simulink library "mbd_s32k_examples"  (Simulink 9.0)
settings: Solver=FixedStepDiscrete  StartTime=0.0  StopTime=10.0  FixedStep=0.1  RelTol=1e-3  EnableMultiTasking=on
InitFcn:
  | mbd_s32k14_consistency_checks(bdroot(gcs));
(part 3 of 3)

== system mbd_s32k_examples/S32K11x MCU Simulink Models/Communications Modules/CAN/CAN_Loopback ==
  Gain : Gain  SaturateOnIntegerOverflow=on  OutDataTypeStr=Inherit: Same as input  ParamDataTypeStr=Inherit: Same as input

== system mbd_s32k_examples/S32K11x MCU Simulink Models/Communications Modules/CAN/CAN_Master_XFER ==
  Gain : Gain  SaturateOnIntegerOverflow=on  OutDataTypeStr=Inherit: Same as input  ParamDataTypeStr=Inherit: Same as input

== system mbd_s32k_examples/S32K11x MCU Simulink Models/Communications Modules/CAN/CAN_Traffic ==
  Gain : Gain  SaturateOnIntegerOverflow=on  OutDataTypeStr=Inherit: Same as input  ParamDataTypeStr=Inherit: Same as input

== system mbd_s32k_examples/S32K11x MCU Simulink Models/Communications Modules/FlexIO/FlexIO_I2C_Master_RX ==
  Gain : Gain  SaturateOnIntegerOverflow=on  OutDataTypeStr=Inherit: Same as input  ParamDataTypeStr=Inherit: Same as input

== system mbd_s32k_examples/S32K11x MCU Simulink Models/Communications Modules/FlexIO/FlexIO_I2C_Master_TX ==
  Gain : Gain  SaturateOnIntegerOverflow=on  OutDataTypeStr=Inherit: Same as input  ParamDataTypeStr=Inherit: Same as input

== system mbd_s32k_examples/S32K11x MCU Simulink Models/Communications Modules/FlexIO/FlexIO_I2C_Slave_RX ==
  Gain : Gain  SaturateOnIntegerOverflow=on  OutDataTypeStr=Inherit: Same as input  ParamDataTypeStr=Inherit: Same as input

== system mbd_s32k_examples/S32K11x MCU Simulink Models/Communications Modules/FlexIO/FlexIO_I2C_Slave_TX ==
  Gain : Gain  SaturateOnIntegerOverflow=on  OutDataTypeStr=Inherit: Same as input  ParamDataTypeStr=Inherit: Same as input

== system mbd_s32k_examples/S32K11x MCU Simulink Models/Communications Modules/FlexIO/FlexIO_SPI_Master_TX ==
  Gain : Gain  SaturateOnIntegerOverflow=on  OutDataTypeStr=Inherit: Same as input  ParamDataTypeStr=Inherit: Same as input

== system mbd_s32k_examples/S32K11x MCU Simulink Models/Communications Modules/FlexIO/FlexIO_SPI_Slave_TX ==
  Gain : Gain  SaturateOnIntegerOverflow=on  OutDataTypeStr=Inherit: Same as input  ParamDataTypeStr=Inherit: Same as input

== system mbd_s32k_examples/S32K11x MCU Simulink Models/Communications Modules/FlexIO/FlexIO_UART_RX ==
  Gain : Gain  SaturateOnIntegerOverflow=on  OutDataTypeStr=Inherit: Same as input  ParamDataTypeStr=Inherit: Same as input

== system mbd_s32k_examples/S32K11x MCU Simulink Models/Communications Modules/FlexIO/FlexIO_UART_TX ==
  Gain : Gain  SaturateOnIntegerOverflow=on  OutDataTypeStr=Inherit: Same as input  ParamDataTypeStr=Inherit: Same as input

== system mbd_s32k_examples/S32K11x MCU Simulink Models/Communications Modules/I2C/I2C_Master_Request ==
  Gain : Gain  SaturateOnIntegerOverflow=on  OutDataTypeStr=Inherit: Same as input  ParamDataTypeStr=Inherit: Same as input

== system mbd_s32k_examples/S32K11x MCU Simulink Models/Communications Modules/I2C/I2C_Master_Send ==
  Gain : Gain  SaturateOnIntegerOverflow=on  OutDataTypeStr=Inherit: Same as input  ParamDataTypeStr=Inherit: Same as input

== system mbd_s32k_examples/S32K11x MCU Simulink Models/Communications Modules/I2C/I2C_Slave_Receive ==
  Gain : Gain  SaturateOnIntegerOverflow=on  OutDataTypeStr=Inherit: Same as input  ParamDataTypeStr=Inherit: Same as input

== system mbd_s32k_examples/S32K11x MCU Simulink Models/Communications Modules/I2C/I2C_Slave_Send ==
  Gain : Gain  SaturateOnIntegerOverflow=on  OutDataTypeStr=Inherit: Same as input  ParamDataTypeStr=Inherit: Same as input

== system mbd_s32k_examples/S32K11x MCU Simulink Models/Communications Modules/SPI/SPI_Master_Slave_Communication ==
  Gain : Gain  SaturateOnIntegerOverflow=on  OutDataTypeStr=Inherit: Same as input  ParamDataTypeStr=Inherit: Same as input

== system mbd_s32k_examples/S32K11x MCU Simulink Models/Communications Modules/Serial/UART_Echo ==
  Gain : Gain  SaturateOnIntegerOverflow=on  OutDataTypeStr=Inherit: Same as input  ParamDataTypeStr=Inherit: Same as input

== system mbd_s32k_examples/S32K11x MCU Simulink Models/Communications Modules/Serial/UART_Hello_World ==
  Gain : Gain  SaturateOnIntegerOverflow=on  OutDataTypeStr=Inherit: Same as input  ParamDataTypeStr=Inherit: Same as input

== system mbd_s32k_examples/S32K14x MCU Simulink Models/AMMCLIB/AMCLIB/AMCLIB_BackEMF_OBSERVER_F16 ==
  Gain : Gain  SaturateOnIntegerOverflow=on  OutDataTypeStr=Inherit: Same as input  ParamDataTypeStr=Inherit: Same as input

== system mbd_s32k_examples/S32K14x MCU Simulink Models/AMMCLIB/AMCLIB/AMCLIB_BackEMF_OBSERVER_F32 ==
  Gain : Gain  SaturateOnIntegerOverflow=on  OutDataTypeStr=Inherit: Same as input  ParamDataTypeStr=Inherit: Same as input

== system mbd_s32k_examples/S32K14x MCU Simulink Models/AMMCLIB/AMCLIB/AMCLIB_BackEMF_OBSERVER_FLT ==
  Gain : Gain  SaturateOnIntegerOverflow=on  OutDataTypeStr=Inherit: Same as input  ParamDataTypeStr=Inherit: Same as input

== system mbd_s32k_examples/S32K14x MCU Simulink Models/AMMCLIB/AMCLIB/AMCLIB_CURRENT_LOOP ==
  Gain : Gain  SaturateOnIntegerOverflow=on  OutDataTypeStr=Inherit: Same as input  ParamDataTypeStr=Inherit: Same as input

== system mbd_s32k_examples/S32K14x MCU Simulink Models/AMMCLIB/AMCLIB/AMCLIB_FW ==
  Gain : Gain  SaturateOnIntegerOverflow=on  OutDataTypeStr=Inherit: Same as input  ParamDataTypeStr=Inherit: Same as input

== system mbd_s32k_examples/S32K14x MCU Simulink Models/AMMCLIB/AMCLIB/AMCLIB_SPEED_LOOP ==
  Gain : Gain  SaturateOnIntegerOverflow=on  OutDataTypeStr=Inherit: Same as input  ParamDataTypeStr=Inherit: Same as input

== system mbd_s32k_examples/S32K14x MCU Simulink Models/AMMCLIB/AMCLIB/AMCLIB_SPEED_LOOP_with_FW ==
  Gain : Gain  SaturateOnIntegerOverflow=on  OutDataTypeStr=Inherit: Same as input  ParamDataTypeStr=Inherit: Same as input

== system mbd_s32k_examples/S32K14x MCU Simulink Models/AMMCLIB/GDFLIB/GDFLIB_FIR ==
  Gain : Gain  SaturateOnIntegerOverflow=on  OutDataTypeStr=Inherit: Same as input  ParamDataTypeStr=Inherit: Same as input

== system mbd_s32k_examples/S32K14x MCU Simulink Models/AMMCLIB/GDFLIB/GDFLIB_IIR1 ==
  Gain : Gain  SaturateOnIntegerOverflow=on  OutDataTypeStr=Inherit: Same as input  ParamDataTypeStr=Inherit: Same as input

== system mbd_s32k_examples/S32K14x MCU Simulink Models/AMMCLIB/GDFLIB/GDFLIB_IIR2 ==
  Gain : Gain  SaturateOnIntegerOverflow=on  OutDataTypeStr=Inherit: Same as input  ParamDataTypeStr=Inherit: Same as input

== system mbd_s32k_examples/S32K14x MCU Simulink Models/AMMCLIB/GDFLIB/GDFLIB_MA ==
  Gain : Gain  SaturateOnIntegerOverflow=on  OutDataTypeStr=Inherit: Same as input  ParamDataTypeStr=Inherit: Same as input

== system mbd_s32k_examples/S32K14x MCU Simulink Models/AMMCLIB/GFLIB/GFLIB_LIMIT ==
  Gain : Gain  SaturateOnIntegerOverflow=on  OutDataTypeStr=Inherit: Same as input  ParamDataTypeStr=Inherit: Same as input

== system mbd_s32k_examples/S32K14x MCU Simulink Models/AMMCLIB/GFLIB/GFLIB_LOG ==
  Gain : Gain  SaturateOnIntegerOverflow=on  OutDataTypeStr=Inherit: Same as input  ParamDataTypeStr=Inherit: Same as input

== system mbd_s32k_examples/S32K14x MCU Simulink Models/AMMCLIB/GFLIB/GFLIB_LUT ==
  Gain : Gain  SaturateOnIntegerOverflow=on  OutDataTypeStr=Inherit: Same as input  ParamDataTypeStr=Inherit: Same as input

== system mbd_s32k_examples/S32K14x MCU Simulink Models/AMMCLIB/GFLIB/GFLIB_MISCELLANEOUS ==
  Gain : Gain  SaturateOnIntegerOverflow=on  OutDataTypeStr=Inherit: Same as input  ParamDataTypeStr=Inherit: Same as input

== system mbd_s32k_examples/S32K14x MCU Simulink Models/AMMCLIB/GFLIB/GFLIB_PIP ==
  Gain : Gain  SaturateOnIntegerOverflow=on  OutDataTypeStr=Inherit: Same as input  ParamDataTypeStr=Inherit: Same as input

== system mbd_s32k_examples/S32K14x MCU Simulink Models/AMMCLIB/GFLIB/GFLIB_PIR ==
  Gain : Gain  SaturateOnIntegerOverflow=on  OutDataTypeStr=Inherit: Same as input  ParamDataTypeStr=Inherit: Same as input

== system mbd_s32k_examples/S32K14x MCU Simulink Models/AMMCLIB/GFLIB/GFLIB_TRIGONOMETRIC ==
  Gain : Gain  SaturateOnIntegerOverflow=on  OutDataTypeStr=Inherit: Same as input  ParamDataTypeStr=Inherit: Same as input

== system mbd_s32k_examples/S32K14x MCU Simulink Models/AMMCLIB/GMCLIB/GMCLIB_FOC_F16 ==
  Gain : Gain  SaturateOnIntegerOverflow=on  OutDataTypeStr=Inherit: Same as input  ParamDataTypeStr=Inherit: Same as input

== system mbd_s32k_examples/S32K14x MCU Simulink Models/AMMCLIB/GMCLIB/GMCLIB_FOC_F32 ==
  Gain : Gain  SaturateOnIntegerOverflow=on  OutDataTypeStr=Inherit: Same as input  ParamDataTypeStr=Inherit: Same as input

== system mbd_s32k_examples/S32K14x MCU Simulink Models/AMMCLIB/GMCLIB/GMCLIB_FOC_FLT ==
  Gain : Gain  SaturateOnIntegerOverflow=on  OutDataTypeStr=Inherit: Same as input  ParamDataTypeStr=Inherit: Same as input

== system mbd_s32k_examples/S32K14x MCU Simulink Models/AMMCLIB/MLIB/MLIB_ABS ==
  Gain : Gain  SaturateOnIntegerOverflow=on  OutDataTypeStr=Inherit: Same as input  ParamDataTypeStr=Inherit: Same as input

== system mbd_s32k_examples/S32K14x MCU Simulink Models/AMMCLIB/MLIB/MLIB_ADD ==
  Gain : Gain  SaturateOnIntegerOverflow=on  OutDataTypeStr=Inherit: Same as input  ParamDataTypeStr=Inherit: Same as input

== system mbd_s32k_examples/S32K14x MCU Simulink Models/AMMCLIB/MLIB/MLIB_CONVERT ==
  Gain : Gain  SaturateOnIntegerOverflow=on  OutDataTypeStr=Inherit: Same as input  ParamDataTypeStr=Inherit: Same as input

== system mbd_s32k_examples/S32K14x MCU Simulink Models/AMMCLIB/MLIB/MLIB_DIV ==
  Gain : Gain  SaturateOnIntegerOverflow=on  OutDataTypeStr=Inherit: Same as input  ParamDataTypeStr=Inherit: Same as input

== system mbd_s32k_examples/S32K14x MCU Simulink Models/AMMCLIB/MLIB/MLIB_MAC ==
  Gain : Gain  SaturateOnIntegerOverflow=on  OutDataTypeStr=Inherit: Same as input  ParamDataTypeStr=Inherit: Same as input

== system mbd_s32k_examples/S32K14x MCU Simulink Models/AMMCLIB/MLIB/MLIB_MUL ==
  Gain : Gain  SaturateOnIntegerOverflow=on  OutDataTypeStr=Inherit: Same as input  ParamDataTypeStr=Inherit: Same as input

== system mbd_s32k_examples/S32K14x MCU Simulink Models/AMMCLIB/MLIB/MLIB_NEGATE ==
  Gain : Gain  SaturateOnIntegerOverflow=on  OutDataTypeStr=Inherit: Same as input  ParamDataTypeStr=Inherit: Same as input

== system mbd_s32k_examples/S32K14x MCU Simulink Models/AMMCLIB/MLIB/MLIB_NORM ==
  Gain : Gain  SaturateOnIntegerOverflow=on  OutDataTypeStr=Inherit: Same as input  ParamDataTypeStr=Inherit: Same as input

== system mbd_s32k_examples/S32K14x MCU Simulink Models/AMMCLIB/MLIB/MLIB_RND ==
  Gain : Gain  SaturateOnIntegerOverflow=on  OutDataTypeStr=Inherit: Same as input  ParamDataTypeStr=Inherit: Same as input

== system mbd_s32k_examples/S32K14x MCU Simulink Models/AMMCLIB/MLIB/MLIB_SHBI ==
  Gain : Gain  SaturateOnIntegerOverflow=on  OutDataTypeStr=Inherit: Same as input  ParamDataTypeStr=Inherit: Same as input

== system mbd_s32k_examples/S32K14x MCU Simulink Models/AMMCLIB/MLIB/MLIB_SHL ==
  Gain : Gain  SaturateOnIntegerOverflow=on  OutDataTypeStr=Inherit: Same as input  ParamDataTypeStr=Inherit: Same as input

== system mbd_s32k_examples/S32K14x MCU Simulink Models/AMMCLIB/MLIB/MLIB_SHR ==
  Gain : Gain  SaturateOnIntegerOverflow=on  OutDataTypeStr=Inherit: Same as input  ParamDataTypeStr=Inherit: Same as input

== system mbd_s32k_examples/S32K14x MCU Simulink Models/AMMCLIB/MLIB/MLIB_SUB ==
  Gain : Gain  SaturateOnIntegerOverflow=on  OutDataTypeStr=Inherit: Same as input  ParamDataTypeStr=Inherit: Same as input

== system mbd_s32k_examples/S32K14x MCU Simulink Models/AMMCLIB/MLIB/MLIB_VMAC ==
  Gain : Gain  SaturateOnIntegerOverflow=on  OutDataTypeStr=Inherit: Same as input  ParamDataTypeStr=Inherit: Same as input

== system mbd_s32k_examples/S32K14x MCU Simulink Models/Communications Modules/CAN/CAN_Echo ==
  Gain : Gain  SaturateOnIntegerOverflow=on  OutDataTypeStr=Inherit: Same as input  ParamDataTypeStr=Inherit: Same as input

== system mbd_s32k_examples/S32K14x MCU Simulink Models/Communications Modules/CAN/CAN_Ecrypted_Master ==
  Gain : Gain  SaturateOnIntegerOverflow=on  OutDataTypeStr=Inherit: Same as input  ParamDataTypeStr=Inherit: Same as input

== system mbd_s32k_examples/S32K14x MCU Simulink Models/Communications Modules/CAN/CAN_Encrypted_Slave ==
  Gain : Gain  SaturateOnIntegerOverflow=on  OutDataTypeStr=Inherit: Same as input  ParamDataTypeStr=Inherit: Same as input

== system mbd_s32k_examples/S32K14x MCU Simulink Models/Communications Modules/CAN/CAN_FD_Master ==
  Gain : Gain  SaturateOnIntegerOverflow=on  OutDataTypeStr=Inherit: Same as input  ParamDataTypeStr=Inherit: Same as input

== system mbd_s32k_examples/S32K14x MCU Simulink Models/Communications Modules/CAN/CAN_FD_Master_XFER ==
  Gain : Gain  SaturateOnIntegerOverflow=on  OutDataTypeStr=Inherit: Same as input  ParamDataTypeStr=Inherit: Same as input

== system mbd_s32k_examples/S32K14x MCU Simulink Models/Communications Modules/CAN/CAN_FD_Slave ==
  Gain : Gain  SaturateOnIntegerOverflow=on  OutDataTypeStr=Inherit: Same as input  ParamDataTypeStr=Inherit: Same as input

== system mbd_s32k_examples/S32K14x MCU Simulink Models/Communications Modules/CAN/CAN_Pretended_Networking ==
  Gain : Gain  SaturateOnIntegerOverflow=on  OutDataTypeStr=Inherit: Same as input  ParamDataTypeStr=Inherit: Same as input

== system mbd_s32k_examples/S32K14x MCU Simulink Models/Communications Modules/CAN/CAN_Traffic ==
  Gain : Gain  SaturateOnIntegerOverflow=on  OutDataTypeStr=Inherit: Same as input  ParamDataTypeStr=Inherit: Same as input

== system mbd_s32k_examples/S32K14x MCU Simulink Models/Communications Modules/CAN/CAN_With_FreeMASTER_over_CAN ==
  Gain : Gain  SaturateOnIntegerOverflow=on  OutDataTypeStr=Inherit: Same as input  ParamDataTypeStr=Inherit: Same as input

== system mbd_s32k_examples/S32K14x MCU Simulink Models/Communications Modules/FlexIO/FlexIO_I2C_Master_RX ==
  Gain : Gain  SaturateOnIntegerOverflow=on  OutDataTypeStr=Inherit: Same as input  ParamDataTypeStr=Inherit: Same as input

== system mbd_s32k_examples/S32K14x MCU Simulink Models/Communications Modules/FlexIO/FlexIO_I2C_Master_TX ==
  Gain : Gain  SaturateOnIntegerOverflow=on  OutDataTypeStr=Inherit: Same as input  ParamDataTypeStr=Inherit: Same as input

== system mbd_s32k_examples/S32K14x MCU Simulink Models/Communications Modules/FlexIO/FlexIO_I2C_Slave_RX ==
  Gain : Gain  SaturateOnIntegerOverflow=on  OutDataTypeStr=Inherit: Same as input  ParamDataTypeStr=Inherit: Same as input

== system mbd_s32k_examples/S32K14x MCU Simulink Models/Communications Modules/FlexIO/FlexIO_I2C_Slave_TX ==
  Gain : Gain  SaturateOnIntegerOverflow=on  OutDataTypeStr=Inherit: Same as input  ParamDataTypeStr=Inherit: Same as input

== system mbd_s32k_examples/S32K14x MCU Simulink Models/Communications Modules/FlexIO/FlexIO_SPI_Master_TX_Blocking ==
  Gain : Gain  SaturateOnIntegerOverflow=on  OutDataTypeStr=Inherit: Same as input  ParamDataTypeStr=Inherit: Same as input

== system mbd_s32k_examples/S32K14x MCU Simulink Models/Communications Modules/FlexIO/FlexIO_SPI_Master_TX_Non_Blocking ==
  Gain : Gain  SaturateOnIntegerOverflow=on  OutDataTypeStr=Inherit: Same as input  ParamDataTypeStr=Inherit: Same as input

== system mbd_s32k_examples/S32K14x MCU Simulink Models/Communications Modules/FlexIO/FlexIO_SPI_Slave_TX_Blocking ==
  Gain : Gain  SaturateOnIntegerOverflow=on  OutDataTypeStr=Inherit: Same as input  ParamDataTypeStr=Inherit: Same as input

== system mbd_s32k_examples/S32K14x MCU Simulink Models/Communications Modules/FlexIO/FlexIO_SPI_Slave_TX_Non_Blocking ==
  Gain : Gain  SaturateOnIntegerOverflow=on  OutDataTypeStr=Inherit: Same as input  ParamDataTypeStr=Inherit: Same as input

== system mbd_s32k_examples/S32K14x MCU Simulink Models/Communications Modules/FlexIO/FlexIO_UART_Hello_World ==
  Gain : Gain  SaturateOnIntegerOverflow=on  OutDataTypeStr=Inherit: Same as input  ParamDataTypeStr=Inherit: Same as input

== system mbd_s32k_examples/S32K14x MCU Simulink Models/Communications Modules/FlexIO/FlexIO_UART_RX ==
  Gain : Gain  SaturateOnIntegerOverflow=on  OutDataTypeStr=Inherit: Same as input  ParamDataTypeStr=Inherit: Same as input

== system mbd_s32k_examples/S32K14x MCU Simulink Models/Communications Modules/FlexIO/FlexIO_UART_TX ==
  Gain : Gain  SaturateOnIntegerOverflow=on  OutDataTypeStr=Inherit: Same as input  ParamDataTypeStr=Inherit: Same as input

== system mbd_s32k_examples/S32K14x MCU Simulink Models/Communications Modules/I2C/I2C_Master_Request ==
  Gain : Gain  SaturateOnIntegerOverflow=on  OutDataTypeStr=Inherit: Same as input  ParamDataTypeStr=Inherit: Same as input

== system mbd_s32k_examples/S32K14x MCU Simulink Models/Communications Modules/I2C/I2C_Master_Send ==
  Gain : Gain  SaturateOnIntegerOverflow=on  OutDataTypeStr=Inherit: Same as input  ParamDataTypeStr=Inherit: Same as input

== system mbd_s32k_examples/S32K14x MCU Simulink Models/Communications Modules/I2C/I2C_Slave_Receive ==
  Gain : Gain  SaturateOnIntegerOverflow=on  OutDataTypeStr=Inherit: Same as input  ParamDataTypeStr=Inherit: Same as input

== system mbd_s32k_examples/S32K14x MCU Simulink Models/Communications Modules/I2C/I2C_Slave_Send ==
  Gain : Gain  SaturateOnIntegerOverflow=on  OutDataTypeStr=Inherit: Same as input  ParamDataTypeStr=Inherit: Same as input

== system mbd_s32k_examples/S32K14x MCU Simulink Models/Communications Modules/SPI/SPI_Master_Slave_Communication ==
  Gain : Gain  SaturateOnIntegerOverflow=on  OutDataTypeStr=Inherit: Same as input  ParamDataTypeStr=Inherit: Same as input

== system mbd_s32k_examples/S32K14x MCU Simulink Models/Communications Modules/Serial/UART_Echo ==
  Gain : Gain  SaturateOnIntegerOverflow=on  OutDataTypeStr=Inherit: Same as input  ParamDataTypeStr=Inherit: Same as input

== system mbd_s32k_examples/S32K14x MCU Simulink Models/Communications Modules/Serial/UART_Hello_World ==
  Gain : Gain  SaturateOnIntegerOverflow=on  OutDataTypeStr=Inherit: Same as input  ParamDataTypeStr=Inherit: Same as input

== system mbd_s32k_examples/S32K14x MCU Simulink Models/Communications Modules/Serial/UART_Relay ==
  Gain : Gain  SaturateOnIntegerOverflow=on  OutDataTypeStr=Inherit: Same as input  ParamDataTypeStr=Inherit: Same as input
